simulink model "diff_eqn"  (R2018a)
settings: Solver=VariableStepAuto  StartTime=0.0  StopTime=10.0  RelTol=1e-3
settings Model: Creator=luan9  LastModifiedBy=luan9

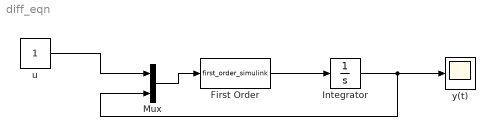
== system diff_eqn ==
  First Order : MATLABFcn  MATLABFcn=first_order_simulink
  Integrator : Integrator  InitialCondition=0.5
  Mux : Mux  Inputs=2
  u : Constant
  y(t) : Scope
  wires:
  First Order/1 -> Integrator/1
  Integrator/1 -> Mux/2, y(t)/1
  u/1 -> Mux/1
  Mux/1 -> First Order/1
